simulink model "old_controller_2013B"  (R2013b)
settings: Solver=ode45  StartTime=0.0  StopTime=sim_run  FixedStep=0.001  RelTol=1e-3
InitFcn:
  | zh = 0.01;
undefined symbols (not defined in the file): Standard_Devices, UDP_Protocol, zh_step
libraries: rtwinlib x6, simulink x2, dspnetwork x2
settings Model: Creator=Lenka  LastModifiedBy=Anony
settings DebuggingCC: UnderspecifiedInitializationDetection=Simplified  MergeDetectMultiDrivingBlocksExec=error  FrameProcessingCompatibilityMsg=error
settings GRTTargetCC: CodeReplacementLibrary=C89/C90 (ANSI)

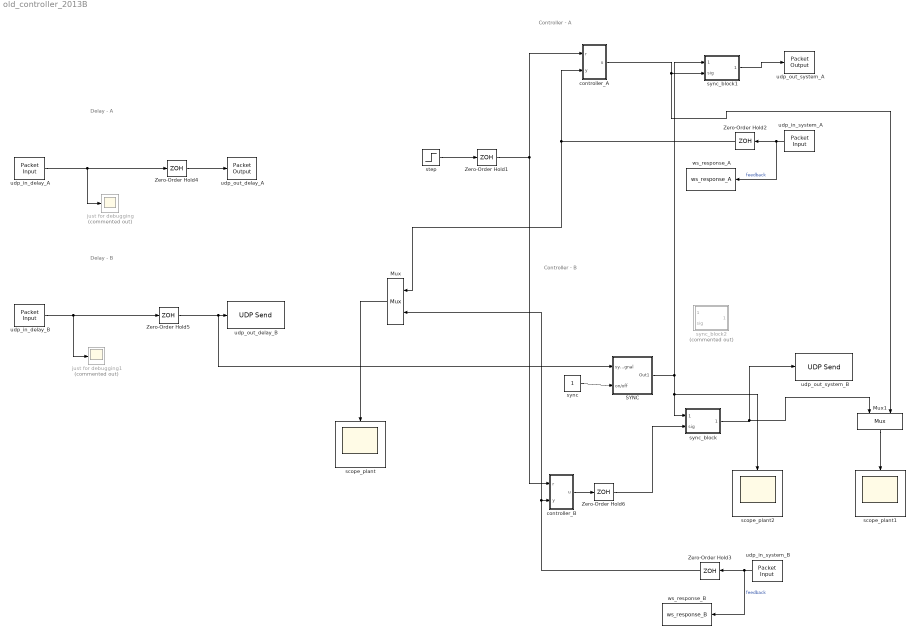
== system old_controller_2013B ==
  note: Controller - B
  note: Controller - A
  note: Delay - A
  note: Delay - B
  Mux : Mux  Inputs=2
  Mux1 : Mux  Inputs=2
  SYNC : Subsystem
  Zero-Order Hold{1..6} (6 alike) : ZeroOrderHold  SampleTime=zh_step
  controller_A : Subsystem
  controller_B : Subsystem
  just for debugging : Scope  Commented=on
      settings: YMin=-10  YMax=10
  just for debugging1 : Scope  Commented=on
      settings: YMin=-10  YMax=10  SaveName=ScopeData2
  scope_plant : Scope
      settings: ShowLegends=on  YMin=-63.375  YMax=570.375
  scope_plant1 : Scope
      settings: ShowLegends=on  YMin=-63.375  YMax=570.375
  scope_plant2 : Scope
      settings: ShowLegends=on  YMin=1  YMax=1  SaveName=ScopeData3
  step : Step  SampleTime=0
  sync : Constant
  sync_block : Subsystem
  sync_block1 : Subsystem
  sync_block2 : Subsystem  Commented=on
  udp_in_delay_A : rtwinlib/Packet Input  SampleTime=0.001  MaxMissedTicks=inf  ShowMissedTicks=off  YieldWhenWaiting=off  DrvName=Standard_Devices/UDP_Protocol  DrvAddress=28000  DrvOptions=[2468394759 28000]  PacketSize=8  DataTypes='double'  ShowReady=off  ShowError=off  PacketID=1  ByteOrder=1  ShowTimestamp=off
      settings: AttributesFormatString=Standard Devices\nUDP Protocol [6978h]
  udp_in_delay_B : rtwinlib/Packet Input  SampleTime=0.001  MaxMissedTicks=inf  ShowMissedTicks=off  YieldWhenWaiting=off  DrvName=Standard_Devices/UDP_Protocol  DrvAddress=28010  DrvOptions=[2468394759 28010]  PacketSize=8  DataTypes='double'  ShowReady=off  ShowError=off  PacketID=1  ByteOrder=1  ShowTimestamp=off
      settings: AttributesFormatString=Standard Devices\nUDP Protocol [6982h]
  udp_in_system_A : rtwinlib/Packet Input  SampleTime=0.001  MaxMissedTicks=inf  ShowMissedTicks=off  YieldWhenWaiting=off  DrvName=Standard_Devices/UDP_Protocol  DrvAddress=28500  DrvOptions=[2468394759 28500]  PacketSize=8  DataTypes='double'  ShowReady=off  ShowError=off  PacketID=1  ByteOrder=1  ShowTimestamp=off
      settings: AttributesFormatString=Standard Devices\nUDP Protocol [6F54h]
  udp_in_system_B : rtwinlib/Packet Input  SampleTime=0.001  MaxMissedTicks=inf  ShowMissedTicks=off  YieldWhenWaiting=off  DrvName=Standard_Devices/UDP_Protocol  DrvAddress=28510  DrvOptions=[2468394759 28510]  PacketSize=8  DataTypes='double'  ShowReady=off  ShowError=off  PacketID=1  ByteOrder=1  ShowTimestamp=off
      settings: AttributesFormatString=Standard Devices\nUDP Protocol [6F54h]
  udp_out_delay_A : rtwinlib/Packet Output  SampleTime=0.01  MaxMissedTicks=inf  ShowMissedTicks=off  YieldWhenWaiting=off  DrvName=Standard_Devices/UDP_Protocol  DrvAddress=27000  DrvOptions=[2468394759 27000]  PacketSize=8  DataTypes='double'  ShowReady=off  ShowError=off  PacketID=1  ByteOrder=1  InitialValue=[]  FinalValue=[]
      settings: AttributesFormatString=Standard Devices\nUDP Protocol [6D60h]
  udp_out_delay_B : dspnetwork/UDP Send  remoteURL='147.32.183.7'  remotePort=27010  localURL='0.0.0.0'  localPortSource=Automatically determine  localPort=27000  sampletime=-1  separateLengthPort=0
  udp_out_system_A : rtwinlib/Packet Output  SampleTime=0.01  MaxMissedTicks=inf  ShowMissedTicks=off  YieldWhenWaiting=off  DrvName=Standard_Devices/UDP_Protocol  DrvAddress=27500  DrvOptions=[2468394759 27500]  PacketSize=8  DataTypes='double'  ShowReady=off  ShowError=off  PacketID=1  ByteOrder=1  InitialValue=[]  FinalValue=[]
      settings: AttributesFormatString=Standard Devices\nUDP Protocol [6B6Ch]
  udp_out_system_B : dspnetwork/UDP Send  remoteURL='147.32.183.7'  remotePort=27510  localURL='0.0.0.0'  localPortSource=Automatically determine  localPort=27000  sampletime=-1  separateLengthPort=0
  ws_response_A : ToWorkspace  VariableName=ws_response_A  SampleTime=zh_step  SaveFormat=Timeseries
  ws_response_B : ToWorkspace  VariableName=ws_response_B  SampleTime=zh_step  SaveFormat=Timeseries
  wires:
  udp_in_system_A/1 -> ws_response_A/1, Zero-Order Hold2/1  "feedback"
  step/1 -> Zero-Order Hold1/1
  udp_in_system_B/1 -> ws_response_B/1, Zero-Order Hold3/1  "feedback"
  Mux/1 -> scope_plant/1
  Zero-Order Hold1/1 -> controller_A/1(r), controller_B/1(r)
  Zero-Order Hold2/1 -> controller_A/2(y), Mux/1
  udp_in_delay_A/1 -> just for debugging/1, Zero-Order Hold4/1
  Zero-Order Hold4/1 -> udp_out_delay_A/1
  udp_in_delay_B/1 -> just for debugging1/1, Zero-Order Hold5/1
  controller_B/1(u) -> Zero-Order Hold6/1
  Zero-Order Hold5/1 -> SYNC/1(sync signal), udp_out_delay_B/1
  sync_block/1(sig out) -> Mux1/1, udp_out_system_B/1
  Zero-Order Hold3/1 -> Mux/2, controller_B/2(y)
  Mux1/1 -> scope_plant1/1
  controller_A/1(u) -> sync_block1/2(sig), Mux1/2
  Zero-Order Hold6/1 -> sync_block/2(sig)
  sync_block1/1(sig out) -> udp_out_system_A/1
  SYNC/1(Out1) -> sync_block1/1(sync_sig), scope_plant2/1, sync_block/1(sync_sig)
  sync/1 -> SYNC/2(on/off)

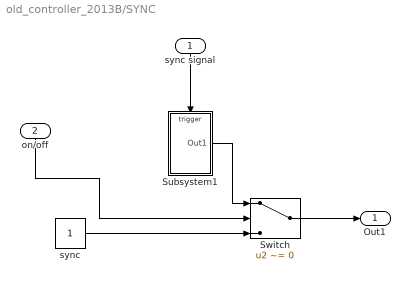
== system old_controller_2013B/SYNC ==
  sync signal : Inport
  on/off : Inport  Port=2
  Subsystem1 : Subsystem
  Switch : Switch  Criteria=u2 ~= 0
  sync : Constant
  Out1 : Outport
  wires:
  sync/1 -> Switch/3
  sync signal/1 -> Subsystem1/Trigger
  Subsystem1/1(Out1) -> Switch/1
  Switch/1 -> Out1/1
  on/off/1 -> Switch/2

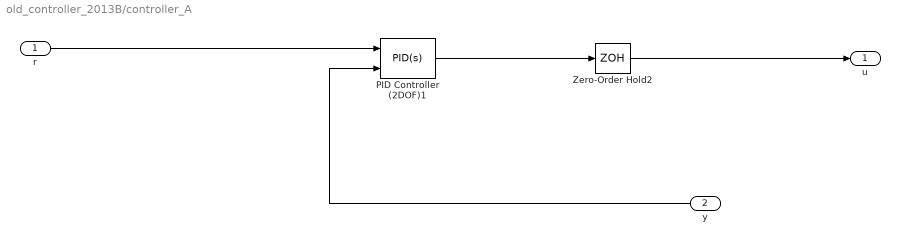
== system old_controller_2013B/controller_A ==
  r : Inport
  y : Inport  Port=2
  PID Controller (2DOF)1 : simulink/Continuous/PID Controller (2DOF)  Controller=PID  TimeDomain=Continuous-time  SampleTime=-1  IntegratorMethod=Forward Euler  FilterMethod=Forward Euler  Form=Parallel  P=6.3799380872686  I=2.12979603411331  D=3.6093223618413  N=48.5068620404972  b=2.39624043732871  c=0.716079145801974  InitialConditionSource=internal  InitialConditionForIntegrator=0  InitialConditionForFilter=0  ExternalReset=none  LimitOutput=off  UpperSaturationLimit=inf  LowerSaturationLimit=-inf  LinearizeAsGain=on  AntiWindupMode=none  Kb=1  TrackingMode=off  Kt=1  PParamMin=[]  PParamMax=[]  IParamMin=[]  IParamMax=[]  DParamMin=[]  DParamMax=[]  NParamMin=[]  NParamMax=[]  bParamMin=[]  bParamMax=[]  cParamMin=[]  cParamMax=[]  KbParamMin=[]  KbParamMax=[]  KtParamMin=[]  KtParamMax=[]  POutMin=[]  POutMax=[]  IOutMin=[]  IOutMax=[]  DOutMin=[]  DOutMax=[]  NOutMin=[]  NOutMax=[]  bOutMin=[]  bOutMax=[]  cOutMin=[]  cOutMax=[]  KbOutMin=[]  KbOutMax=[]  KtOutMin=[]  KtOutMax=[]  IntegratorOutMin=[]  IntegratorOutMax=[]  FilterOutMin=[]  FilterOutMax=[]  SumOutMin=[]  SumOutMax=[]  Sum1OutMin=[]  Sum1OutMax=[]  Sum2OutMin=[]  Sum2OutMax=[]  Sum3OutMin=[]  Sum3OutMax=[]  SumI1OutMin=[]  SumI1OutMax=[]  SumI2OutMin=[]  SumI2OutMax=[]  SumI3OutMin=[]  SumI3OutMax=[]  SumDOutMin=[]  SumDOutMax=[]  SaturationOutMin=[]  SaturationOutMax=[]  IntegratorContinuousStateAttributes=''  IntegratorStateMustResolveToSignalObject=off  IntegratorRTWStateStorageClass=Auto  FilterContinuousStateAttributes=''  FilterStateMustResolveToSignalObject=off  FilterRTWStateStorageClass=Auto
  Zero-Order Hold2 : ZeroOrderHold  SampleTime=zh_step
  u : Outport
  wires:
  r/1 -> PID Controller (2DOF)1/1
  y/1 -> PID Controller (2DOF)1/2
  Zero-Order Hold2/1 -> u/1
  PID Controller (2DOF)1/1 -> Zero-Order Hold2/1

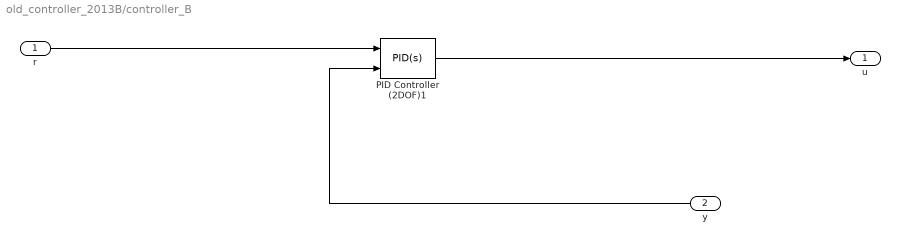
== system old_controller_2013B/controller_B ==
  r : Inport
  y : Inport  Port=2
  PID Controller (2DOF)1 : simulink/Continuous/PID Controller (2DOF)  Controller=PID  TimeDomain=Continuous-time  SampleTime=-1  IntegratorMethod=Forward Euler  FilterMethod=Forward Euler  Form=Parallel  P=6.3799380872686  I=2.12979603411331  D=3.6093223618413  N=48.5068620404972  b=2.39624043732871  c=0.716079145801974  InitialConditionSource=internal  InitialConditionForIntegrator=0  InitialConditionForFilter=0  ExternalReset=none  LimitOutput=off  UpperSaturationLimit=inf  LowerSaturationLimit=-inf  LinearizeAsGain=on  AntiWindupMode=none  Kb=1  TrackingMode=off  Kt=1  PParamMin=[]  PParamMax=[]  IParamMin=[]  IParamMax=[]  DParamMin=[]  DParamMax=[]  NParamMin=[]  NParamMax=[]  bParamMin=[]  bParamMax=[]  cParamMin=[]  cParamMax=[]  KbParamMin=[]  KbParamMax=[]  KtParamMin=[]  KtParamMax=[]  POutMin=[]  POutMax=[]  IOutMin=[]  IOutMax=[]  DOutMin=[]  DOutMax=[]  NOutMin=[]  NOutMax=[]  bOutMin=[]  bOutMax=[]  cOutMin=[]  cOutMax=[]  KbOutMin=[]  KbOutMax=[]  KtOutMin=[]  KtOutMax=[]  IntegratorOutMin=[]  IntegratorOutMax=[]  FilterOutMin=[]  FilterOutMax=[]  SumOutMin=[]  SumOutMax=[]  Sum1OutMin=[]  Sum1OutMax=[]  Sum2OutMin=[]  Sum2OutMax=[]  Sum3OutMin=[]  Sum3OutMax=[]  SumI1OutMin=[]  SumI1OutMax=[]  SumI2OutMin=[]  SumI2OutMax=[]  SumI3OutMin=[]  SumI3OutMax=[]  SumDOutMin=[]  SumDOutMax=[]  SaturationOutMin=[]  SaturationOutMax=[]  IntegratorContinuousStateAttributes=''  IntegratorStateMustResolveToSignalObject=off  IntegratorRTWStateStorageClass=Auto  FilterContinuousStateAttributes=''  FilterStateMustResolveToSignalObject=off  FilterRTWStateStorageClass=Auto
  u : Outport
  wires:
  PID Controller (2DOF)1/1 -> u/1
  y/1 -> PID Controller (2DOF)1/2
  r/1 -> PID Controller (2DOF)1/1

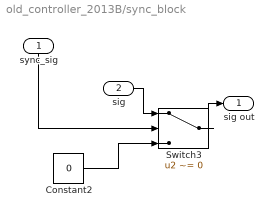
== system old_controller_2013B/sync_block ==
  sync_sig : Inport
  sig : Inport  Port=2
  Constant2 : Constant  Value=0
  Switch3 : Switch  Criteria=u2 ~= 0
  sig out : Outport
  wires:
  Constant2/1 -> Switch3/3
  sig/1 -> Switch3/1
  Switch3/1 -> sig out/1
  sync_sig/1 -> Switch3/2

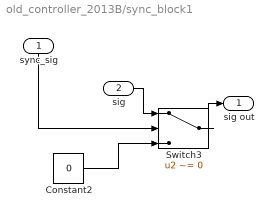
== system old_controller_2013B/sync_block1 ==
  sync_sig : Inport
  sig : Inport  Port=2
  Constant2 : Constant  Value=0
  Switch3 : Switch  Criteria=u2 ~= 0
  sig out : Outport
  wires:
  sync_sig/1 -> Switch3/2
  Switch3/1 -> sig out/1
  sig/1 -> Switch3/1
  Constant2/1 -> Switch3/3

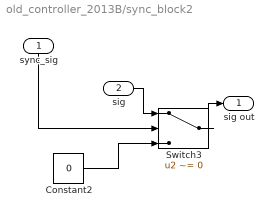
== system old_controller_2013B/sync_block2 ==
  sync_sig : Inport
  sig : Inport  Port=2
  Constant2 : Constant  Value=0
  Switch3 : Switch  Criteria=u2 ~= 0
  sig out : Outport
  wires:
  sync_sig/1 -> Switch3/2
  Switch3/1 -> sig out/1
  sig/1 -> Switch3/1
  Constant2/1 -> Switch3/3

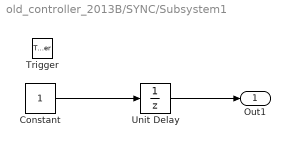
== system old_controller_2013B/SYNC/Subsystem1 ==
  Trigger : TriggerPort  PortDimensions=1
  Constant : Constant
  Unit Delay : UnitDelay  SampleTime=-1
  Out1 : Outport
  wires:
  Unit Delay/1 -> Out1/1
  Constant/1 -> Unit Delay/1
